simulink model "final_problema_3_sim2021"  (R2023b)
settings: Solver=VariableStepAuto  StartTime=0.0  StopTime=100  RelTol=1e-3
libraries: cstblocks x1
settings Model: Creator=cgbri  LastModifiedBy=Maxi
settings RTWCC: GPUComputeCapability=5.0

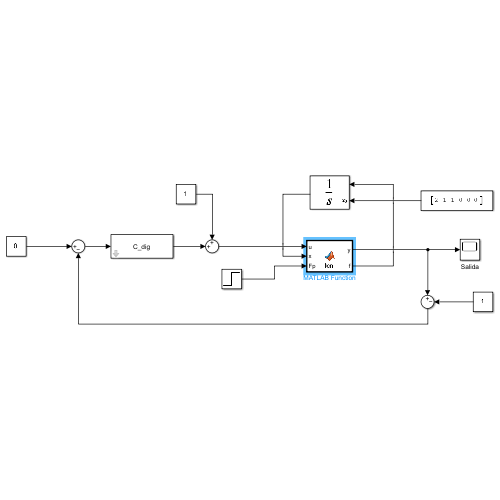
[thumbnail: Simulink's stored preview of the top-level diagram]
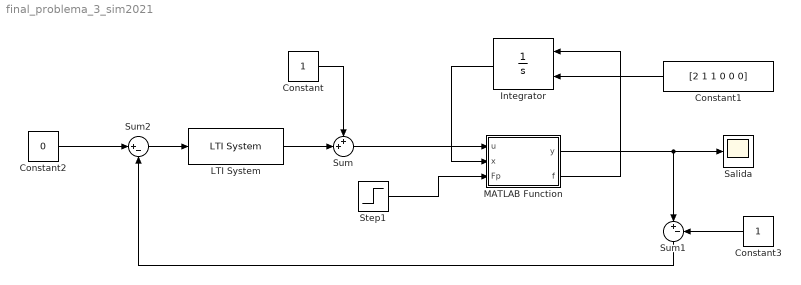
== system final_problema_3_sim2021 ==
  Constant : Constant
  Constant1 : Constant  Value=[2 1 1 0 0 0]
  Constant2 : Constant  Value=0
  Constant3 : Constant
  Integrator : Integrator  InitialConditionSource=external
  LTI System : cstblocks/LTI System  sys=C_dig  IC=[]  PadeOrder=0
  MATLAB Function : MATLAB Function  TreatAsAtomicUnit=on
  Salida : Scope
  Step1 : Step  After=0.1  SampleTime=0
  Sum : Sum  Inputs=++|
  Sum1 : Sum  Inputs=|+-
  Sum2 : Sum  Inputs=|+-
  wires:
  Integrator/1 -> MATLAB Function/2(x)
  MATLAB Function/2(f) -> Integrator/1
  Constant1/1 -> Integrator/2
  Step1/1 -> MATLAB Function/3(Fp)
  MATLAB Function/1(y) -> Sum1/1, Salida/1
  Sum/1 -> MATLAB Function/1(u)
  Constant/1 -> Sum/1
  Constant3/1 -> Sum1/2
  Sum1/1 -> Sum2/2
  LTI System/1 -> Sum/2
  Sum2/1 -> LTI System/1
  Constant2/1 -> Sum2/1

== matlab function final_problema_3_sim2021/MATLAB Function ==
  data: u input; y output; x input; f output; Fp input
function [y,f] = fcn(u, x, Fp)
    %Constantes
    p = 0.02;
    
    %Ecuaciones no lineales
    F1 = ( x(3) - sqrt(x(1)-x(2)) )/power(x(1), 2);
    F2 = ( sqrt(x(1)-x(2)) - sqrt(x(2)) + Fp )/power(x(2), 2);
    F3 = p*u-p*x(3);
    
    y = x(2);
    f = [F1 F2 F3];
